simulink model "PPS_Model"  (Simulink 7.6)
settings: Solver=FixedStepDiscrete  SolverMode=SingleTasking  StartTime=0.0  StopTime=inf  FixedStep=1/100  RelTol=1e-3
undefined symbols (not defined in the file): dfreq, gray, nbboxout, Rec, SDTV, strel
libraries: simulink x21, viptextngfix x15, simulink_extras x3, vipconversions x3, vipsnks x2, vipstatistics x1, vipmorphops x1, vipanalysis x1
(part 1 of 2)
settings Model: Creator=Krzysztof  LastModifiedBy=MarcinB  BufferReuse=off
settings DataIOCC: SaveOutput=off  SaveTime=off
settings OptimizationCC: InlineParams=on  OptimizeBlockIOStorage=off  BufferReuse=off  ExpressionFolding=off  LocalBlockOutputs=off  SimCompilerOptimization=On
settings DebuggingCC: ReadBeforeWriteMsg=DisableAll  WriteAfterWriteMsg=DisableAll  WriteAfterReadMsg=DisableAll  SolverPrmCheckMsg=none  MultiTaskDSMMsg=none  SigSpecEnsureSampleTimeMsg=none  ParameterPrecisionLossMsg=none  UnknownTsInhSupMsg=none
settings ModelReferenceCC: ModelReferenceNumInstancesAllowed=Single
settings SFSimCC: SimParseCustomCode=off

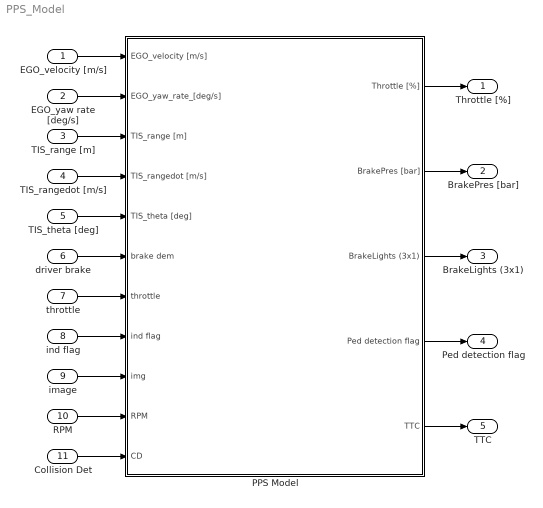
== system PPS_Model ==
  EGO_velocity [m/s] : Inport
  EGO_yaw rate [deg/s] : Inport  Port=2
  TIS_range [m] : Inport  Port=3
  TIS_rangedot [m/s] : Inport  Port=4
  TIS_theta [deg] : Inport  Port=5
  driver brake : Inport  Port=6
  throttle : Inport  Port=7
  ind flag : Inport  Port=8
  image : Inport  Port=9
  RPM : Inport  Port=10
  Collision Det : Inport  Port=11
  PPS Model : Subsystem  mask(PPS Model){MaxSpeed=70, MaxBrakePressure=150, BrakeDelay=100, LaneWidth=3.5, TISMaxRange=40, TISMaxTheta=60, TISfreq=25, TISdet=32, Camfreq=50, Mainfreq=100, DisplaySwitch=on, DisplayFreq=25, RadarSwitch=on, RadarFreq=25}
      mask prompts: MaxSpeed "Vehicle cut-off speed [km/h]"; MaxBrakePressure "Maximum value of braking pressure available [bar]"; BrakeDelay "Braking system delay [ms]"; LaneWidth "Lane width [m]"; TISMaxRange "TIS maximum range [m]"; TISMaxTheta "TIS maximum theta [deg]"; TISfreq "TIS frequency [Hz]"; TISdet "Max. number of Radar detected objects [-]"; Camfreq "Camera frequency [Hz]"; Mainfreq "Compilation sheet frequency [Hz]"; DisplaySwitch "Show EGO parameters visualization"; DisplayFreq "EGO parameters visualization frequency [Hz]"; RadarSwitch "Show radar visualization"; RadarFreq "Radar frequency [Hz]"
      mask help: PreScan Experiment and Pedestrian Protection System parameters
      mask Help: eval('openHelp(8130)')
      mask CallbackString:
      | ||||||||||en = get_param(gcb,'MaskEnables');
      | switch get_param(gcb, 'DisplaySwitch')
      |     case 'off'
      |         en{12} = 'off';
      |     case 'on'
      |         en{12} = 'on';
      | end
      | set_param(gcb,'MaskEnables',en);
      | clear en;||en = get_param(gcb,'MaskEnables');
      | switch get_param(gcb, 'RadarSwitch')
      |     case 'off'
      |         en{14} = 'off';
      |     case 'on'
      |         en{14} = 'on';
      | end
      | set_param(gcb,'MaskEnables',en);
      | clear en;|
  Throttle [%] : Outport
  BrakePres [bar] : Outport  Port=2
  BrakeLights (3x1) : Outport  Port=3
  Ped detection flag : Outport  Port=4
  TTC : Outport  Port=5
  wires:
  EGO_velocity [m/s]/1 -> PPS Model/1(EGO_velocity [m/s])
  EGO_yaw rate [deg/s]/1 -> PPS Model/2(EGO_yaw_rate_[deg/s])
  TIS_range [m]/1 -> PPS Model/3(TIS_range [m])
  TIS_rangedot [m/s]/1 -> PPS Model/4(TIS_rangedot [m/s])
  TIS_theta [deg]/1 -> PPS Model/5(TIS_theta [deg])
  throttle/1 -> PPS Model/7(throttle)
  ind flag/1 -> PPS Model/8(ind flag)
  image/1 -> PPS Model/9(img)
  PPS Model/1(Throttle [%]) -> Throttle [%]/1
  PPS Model/2(BrakePres [bar]) -> BrakePres [bar]/1
  PPS Model/3(BrakeLights (3x1)) -> BrakeLights (3x1)/1
  PPS Model/5(TTC) -> TTC/1
  driver brake/1 -> PPS Model/6(brake dem)
  RPM/1 -> PPS Model/10(RPM)
  Collision Det/1 -> PPS Model/11(CD)
  PPS Model/4(Ped detection flag) -> Ped detection flag/1

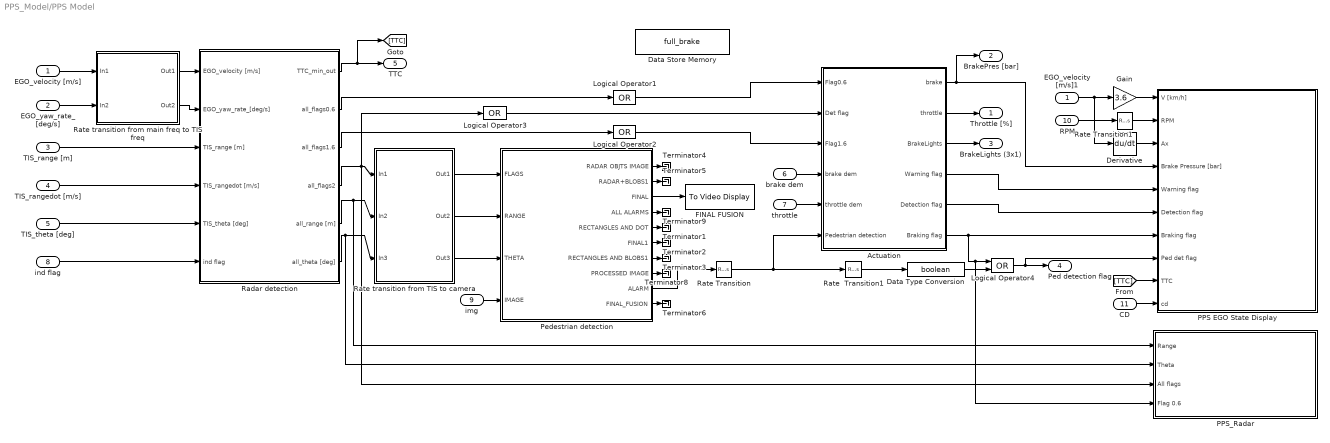
== system PPS_Model/PPS Model ==
  EGO_velocity [m/s] : Inport
  EGO_yaw_rate_[deg/s] : Inport  Port=2  SampleTime=1/Mainfreq
  TIS_range [m] : Inport  Port=3  PortDimensions=TISdet  SampleTime=1/TISfreq
  TIS_rangedot [m/s] : Inport  Port=4  PortDimensions=TISdet  SampleTime=1/TISfreq
  TIS_theta [deg] : Inport  Port=5  PortDimensions=TISdet  SampleTime=1/TISfreq
  brake dem : Inport  Port=6  SampleTime=[0,0]
  throttle : Inport  Port=7  SampleTime=[0,0]
  ind flag : Inport  Port=8  SampleTime=1/TISfreq
  img : Inport  Port=9  PortDimensions=[375 500]  SampleTime=1/Camfreq
  RPM : Inport  Port=10
  CD : Inport  Port=11
  Actuation : Subsystem
  Data Store Memory : DataStoreMemory  DataStoreName=full_brake  ReadBeforeWriteMsg=warning  WriteAfterWriteMsg=warning  WriteAfterReadMsg=warning
  Data Type Conversion : DataTypeConversion  OutDataTypeStr=boolean
  Derivative : Derivative
  EGO_velocity [m/s]1 : InportShadow  Port=1
  FINAL FUSION : vipsnks/To Video Display  DialogControllerArgs=DataTag0  inputType=Obsolete  imagePorts=One multidimensional signal  OutputDevice=On-screen video monitor  fullScreen=off  videoWindowX=530  videoWindowY=74  saveWindowSize=off  videoWindowWidth=500  videoWindowHeight=375  dataOrg=Column-major  openAtMdlStart=on  isWindowOpen=on
  Gain : Gain  Gain=3.6
  Logical Operator1 : Logic  Operator=OR  Inputs=1  AllPortsSameDT=off  OutDataTypeStr=boolean
  Logical Operator2 : Logic  Operator=OR  Inputs=1  AllPortsSameDT=off  OutDataTypeStr=boolean
  Logical Operator3 : Logic  Operator=OR  Inputs=1  AllPortsSameDT=off  OutDataTypeStr=boolean
  Logical Operator4 : Logic  Operator=OR  AllPortsSameDT=off  OutDataTypeStr=boolean
  PPS EGO State Display : Subsystem
  PPS_Radar : Subsystem
  Pedestrian detection : Subsystem
  Radar detection : Subsystem
  Rate  Transition1 : RateTransition  Integrity=off  Deterministic=off  OutPortSampleTime=1/min(TISfreq,Camfreq)
  Rate Transition : RateTransition  Integrity=off  Deterministic=off  OutPortSampleTime=[0,0]
  Rate Transition1 : RateTransition  Integrity=off  Deterministic=off  OutPortSampleTime=1/Mainfreq
  Rate transition from TIS to camera : Subsystem
  Rate transition from main freq to TIS freq : Subsystem
  Terminator{1..6,8..9} (8 alike) : Terminator
  Throttle [%] : Outport
  BrakePres [bar] : Outport  Port=2
  BrakeLights (3x1) : Outport  Port=3
  Ped detection flag : Outport  Port=4  PortDimensions=1
  TTC : Outport  Port=5
  wires:
  TIS_range [m]/1 -> Radar detection/3(TIS_range [m])
  TIS_rangedot [m/s]/1 -> Radar detection/4(TIS_rangedot [m/s])
  TIS_theta [deg]/1 -> Radar detection/5(TIS_theta [deg])
  ind flag/1 -> Radar detection/6(ind flag)
  EGO_velocity [m/s]/1 -> Rate transition from main freq to TIS freq/1(In1)
  EGO_yaw_rate_[deg/s]/1 -> Rate transition from main freq to TIS freq/2(In2)
  Rate transition from main freq to TIS freq/1(Out1) -> Radar detection/1(EGO_velocity [m/s])
  Rate transition from main freq to TIS freq/2(Out2) -> Radar detection/2(EGO_yaw_rate_[deg/s])
  throttle/1 -> Actuation/5(throttle dem)
  brake dem/1 -> Actuation/4(brake dem)
  Radar detection/1(TTC_min_out) -> TTC/1, [TTC]
  Radar detection/2(all_flags0.6) -> Logical Operator1/1
  Rate Transition/1 -> Actuation/6(Pedestrian detection), Rate  Transition1/1
  Rate  Transition1/1 -> Data Type Conversion/1
  Radar detection/4(all_flags2) -> Rate transition from TIS to camera/1(In1), Logical Operator3/1, PPS_Radar/3(All flags)
  Radar detection/5(all_range [m]) -> Rate transition from TIS to camera/2(In2), PPS_Radar/1(Range)
  Radar detection/6(all_theta [deg]) -> Rate transition from TIS to camera/3(In3), PPS_Radar/2(Theta)
  Radar detection/3(all_flags1.6) -> Logical Operator2/1
  Actuation/1(brake) -> BrakePres [bar]/1, PPS EGO State Display/4(Brake Pressure [bar])
  Actuation/2(throttle) -> Throttle [%]/1
  Actuation/3(BrakeLights) -> BrakeLights (3x1)/1
  Actuation/6(Braking flag) -> PPS EGO State Display/7(Braking flag), Logical Operator4/1, PPS_Radar/4(Flag 0.6)
  Pedestrian detection/8(PROCESSED IMAGE) -> Terminator8/1
  Pedestrian detection/4(ALL ALARMS) -> Terminator9/1
  Pedestrian detection/5(RECTANGLES AND DOT) -> Terminator1/1
  Pedestrian detection/7(RECTANGLES AND BLOBS1) -> Terminator3/1
  Pedestrian detection/2(RADAR+BLOBS1) -> Terminator5/1
  Pedestrian detection/1(RADAR OBJTS IMAGE) -> Terminator4/1
  Pedestrian detection/10(FINAL_FUSION) -> Terminator6/1
  img/1 -> Pedestrian detection/4(IMAGE)
  Pedestrian detection/3(FINAL) -> FINAL FUSION/1
  Pedestrian detection/9(ALARM) -> Rate Transition/1
  Pedestrian detection/6(FINAL1) -> Terminator2/1
  Rate transition from TIS to camera/1(Out1) -> Pedestrian detection/1(FLAGS)
  Rate transition from TIS to camera/2(Out2) -> Pedestrian detection/2(RANGE)
  Rate transition from TIS to camera/3(Out3) -> Pedestrian detection/3(THETA)
  Logical Operator1/1 -> Actuation/1(Flag0.6)
  Logical Operator2/1 -> Actuation/3(Flag1.6)
  Data Type Conversion/1 -> Logical Operator4/2
  Logical Operator4/1 -> Ped detection flag/1, PPS EGO State Display/8(Ped det flag)
  Logical Operator3/1 -> Actuation/2(Det flag)
  EGO_velocity [m/s]1/1 -> Gain/1, Derivative/1
  Gain/1 -> PPS EGO State Display/1(V [km/h])
  RPM/1 -> Rate Transition1/1
  Derivative/1 -> PPS EGO State Display/3(Ax)
  CD/1 -> PPS EGO State Display/10(cd)
  [TTC] -> PPS EGO State Display/9(TTC)
  Actuation/4(Warning flag) -> PPS EGO State Display/5(Warning flag)
  Actuation/5(Detection flag) -> PPS EGO State Display/6(Detection flag)
  Rate Transition1/1 -> PPS EGO State Display/2(RPM)

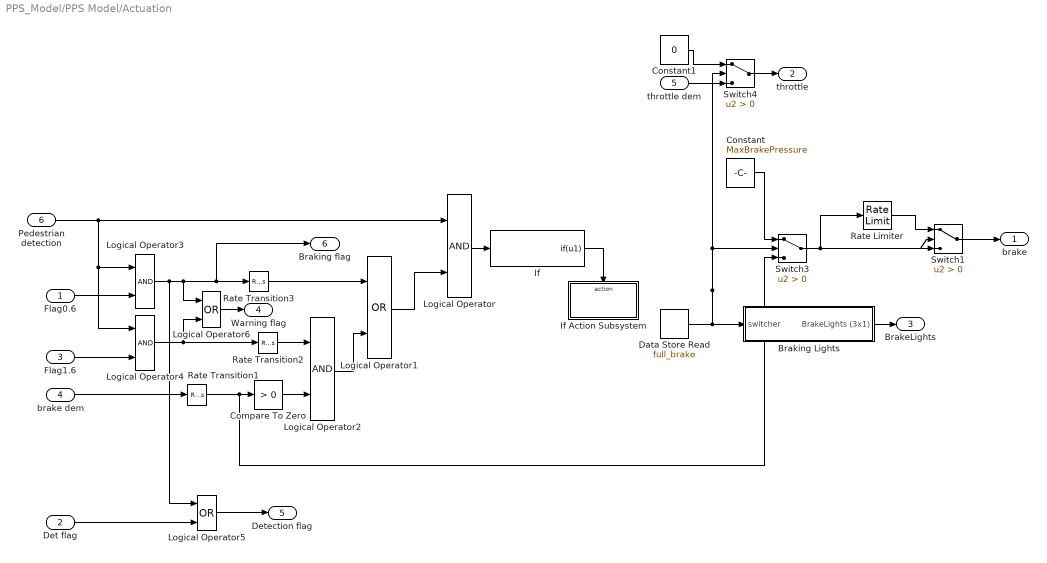
== system PPS_Model/PPS Model/Actuation ==
  Flag0.6 : Inport
  Det flag : Inport  Port=2
  Flag1.6 : Inport  Port=3
  brake dem : Inport  Port=4
  throttle dem : Inport  Port=5
  Pedestrian detection : Inport  Port=6
  Braking Lights : Subsystem
  Compare To Zero : simulink/Logic and Bit Operations/Compare To Zero  SystemSampleTime=-1  relop=>  LogicOutDataTypeMode=uint8
  Constant : Constant  Value=MaxBrakePressure  SampleTime=[0,0]
  Constant1 : Constant  Value=0  SampleTime=[0,0]
  Data Store Read : DataStoreRead  DataStoreName=full_brake  SampleTime=1/Mainfreq
  If : If  IfExpression=u1  ShowElse=off
  If Action Subsystem : Subsystem  TreatAsAtomicUnit=on
  Logical Operator : Logic  AllPortsSameDT=off  OutDataTypeStr=boolean  SampleTime=[0,0]
  Logical Operator1 : Logic  Operator=OR  AllPortsSameDT=off  OutDataTypeStr=boolean  SampleTime=[0,0]
  Logical Operator2 : Logic  AllPortsSameDT=off  OutDataTypeStr=boolean  SampleTime=[0,0]
  Logical Operator3 : Logic  AllPortsSameDT=off  OutDataTypeStr=boolean  SampleTime=1/TISfreq
  Logical Operator4 : Logic  AllPortsSameDT=off  OutDataTypeStr=boolean  SampleTime=1/TISfreq
  Logical Operator5 : Logic  Operator=OR  AllPortsSameDT=off  OutDataTypeStr=boolean  SampleTime=1/TISfreq
  Logical Operator6 : Logic  Operator=OR  AllPortsSameDT=off  OutDataTypeStr=boolean  SampleTime=1/TISfreq
  Rate Limiter : RateLimiter  RisingSlewLimit=1000*0.9*MaxBrakePressure/BrakeDelay  FallingSlewLimit=-inf  SampleTimeMode=inherited
  Rate Transition1 : RateTransition  Integrity=off  OutPortSampleTime=[0,0]
  Rate Transition2 : RateTransition  Integrity=off  OutPortSampleTime=[0,0]
  Rate Transition3 : RateTransition  Integrity=off  OutPortSampleTime=[0,0]
  Switch1 : Switch  Criteria=u2 > Threshold  SampleTime=[0,0]
  Switch3 : Switch  Criteria=u2 > Threshold  SampleTime=[0,0]
  Switch4 : Switch  Criteria=u2 > Threshold  SampleTime=[0,0]
  brake : Outport  SampleTime=[0,0]
  throttle : Outport  Port=2  SampleTime=[0,0]
  BrakeLights : Outport  Port=3  SampleTime=1/Mainfreq
  Warning flag : Outport  Port=4
  Detection flag : Outport  Port=5
  Braking flag : Outport  Port=6
  wires:
  Pedestrian detection/1 -> Logical Operator3/1, Logical Operator4/1, Logical Operator/1
  Logical Operator1/1 -> Logical Operator/2
  Logical Operator2/1 -> Logical Operator1/2
  Compare To Zero/1 -> Logical Operator2/2
  Constant/1 -> Switch3/1
  Constant1/1 -> Switch4/1
  Switch4/1 -> throttle/1
  throttle dem/1 -> Switch4/3
  Braking Lights/1(BrakeLights (3x1)) -> BrakeLights/1
  brake dem/1 -> Rate Transition1/1
  Rate Transition1/1 -> Compare To Zero/1, Switch3/3
  Rate Transition2/1 -> Logical Operator2/1
  Rate Transition3/1 -> Logical Operator1/1
  Switch3/1 -> Switch1/3, Rate Limiter/1
  Rate Limiter/1 -> Switch1/1
  Switch1/1 -> brake/1
  Logical Operator3/1 -> Rate Transition3/1, Braking flag/1, Logical Operator6/1, Logical Operator5/1
  Logical Operator4/1 -> Rate Transition2/1, Logical Operator6/2
  Flag0.6/1 -> Logical Operator3/2
  Flag1.6/1 -> Logical Operator4/2
  Logical Operator6/1 -> Warning flag/1
  Det flag/1 -> Logical Operator5/2
  Logical Operator5/1 -> Detection flag/1
  Logical Operator/1 -> If/1
  Data Store Read/1 -> Braking Lights/1(switcher), Switch3/2, Switch1/2, Switch4/2
  If/1 -> If Action Subsystem/Action

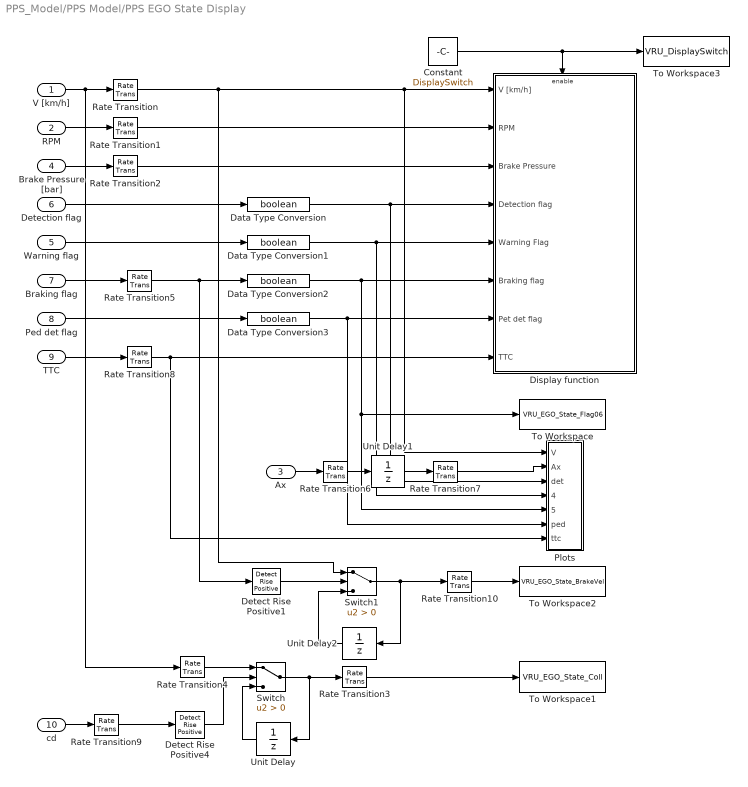
== system PPS_Model/PPS Model/PPS EGO State Display ==
  V [km/h] : Inport
  RPM : Inport  Port=2
  Ax : Inport  Port=3  SampleTime=[0,0]
  Brake Pressure [bar] : Inport  Port=4
  Warning flag : Inport  Port=5  OutDataTypeStr=boolean
  Detection flag : Inport  Port=6  OutDataTypeStr=boolean
  Braking flag : Inport  Port=7  OutDataTypeStr=boolean
  Ped det flag : Inport  Port=8  OutDataTypeStr=boolean
  TTC : Inport  Port=9
  cd : Inport  Port=10  OutDataTypeStr=boolean
  Constant : Constant  Value=DisplaySwitch
  Data Type Conversion{,1..3} (4 alike) : DataTypeConversion  OutDataTypeStr=boolean
  Detect Rise Positive1 : simulink/Logic and Bit Operations/Detect Rise Positive  SystemSampleTime=-1  vinit=0
  Detect Rise Positive4 : simulink/Logic and Bit Operations/Detect Rise Positive  SystemSampleTime=-1  vinit=0
  Display function : Subsystem
  Plots : Subsystem
      mask Description:
      | The block calls functions:
      | * PPS_Speed_Profile
      | * PPS_TTC_Profile
      | to generate plots at the end of the simulation.
      | See stop callback of the block for more details.
  Rate Transition{,1..2,5,7..8} (6 alike) : RateTransition  Integrity=off  OutPortSampleTime=1/DisplayFreq
  Rate Transition10 : RateTransition  Integrity=off  OutPortSampleTime=[0,0]
  Rate Transition3 : RateTransition  Integrity=off  OutPortSampleTime=[0,0]
  Rate Transition4 : RateTransition  Integrity=off  OutPortSampleTime=1/Mainfreq
  Rate Transition6 : RateTransition  Integrity=off  OutPortSampleTimeOpt=Inherit  OutPortSampleTime=1/dfreq
  Rate Transition9 : RateTransition  Integrity=off  OutPortSampleTime=1/Mainfreq
  Switch : Switch  Criteria=u2 > Threshold  SampleTime=1/Mainfreq
  Switch1 : Switch  Criteria=u2 > Threshold  SampleTime=1/Mainfreq
  To Workspace : ToWorkspace  VariableName=VRU_EGO_State_Flag06  SampleTime=-1  SaveFormat=Array
      settings: MaxDataPoints=1
  To Workspace1 : ToWorkspace  VariableName=VRU_EGO_State_Coll  SampleTime=1/Mainfreq  SaveFormat=Array
      settings: MaxDataPoints=1
  To Workspace2 : ToWorkspace  VariableName=VRU_EGO_State_BrakeVel  SampleTime=1/Mainfreq  SaveFormat=Array
      settings: MaxDataPoints=1
  To Workspace3 : ToWorkspace  VariableName=VRU_DisplaySwitch  SampleTime=-1  SaveFormat=Array
      settings: MaxDataPoints=1
  Unit Delay : UnitDelay  SampleTime=1/Mainfreq
  Unit Delay1 : UnitDelay  SampleTime=-1
  Unit Delay2 : UnitDelay  SampleTime=1/Mainfreq
  wires:
  RPM/1 -> Rate Transition1/1
  Brake Pressure [bar]/1 -> Rate Transition2/1
  V [km/h]/1 -> Rate Transition/1, Rate Transition4/1
  Warning flag/1 -> Data Type Conversion1/1
  Ped det flag/1 -> Data Type Conversion3/1
  TTC/1 -> Rate Transition8/1
  Detection flag/1 -> Data Type Conversion/1
  Rate Transition/1 -> Display function/1(V [km/h]), Plots/1(V), Switch1/1
  Rate Transition1/1 -> Display function/2(RPM)
  Rate Transition3/1 -> To Workspace1/1
  cd/1 -> Rate Transition9/1
  Switch/1 -> Unit Delay/1, Rate Transition3/1
  Unit Delay/1 -> Switch/3
  Rate Transition4/1 -> Switch/1
  Detect Rise Positive4/1 -> Switch/2
  Braking flag/1 -> Rate Transition5/1
  Rate Transition5/1 -> Data Type Conversion2/1, Detect Rise Positive1/1
  Ax/1 -> Rate Transition6/1
  Unit Delay1/1 -> Rate Transition7/1
  Rate Transition6/1 -> Unit Delay1/1
  Rate Transition2/1 -> Display function/3(Brake Pressure)
  Rate Transition7/1 -> Plots/2(Ax)
  Rate Transition8/1 -> Plots/7(ttc), Display function/8(TTC)
  Rate Transition9/1 -> Detect Rise Positive4/1
  Data Type Conversion3/1 -> Plots/6(ped), Display function/7(Pet det flag)
  Data Type Conversion2/1 -> Plots/5(brake), To Workspace/1, Display function/6(Braking flag)
  Data Type Conversion1/1 -> Plots/4(warn), Display function/5(Warning Flag)
  Data Type Conversion/1 -> Plots/3(det), Display function/4(Detection flag)
  Constant/1 -> Display function/Enable, To Workspace3/1
  Detect Rise Positive1/1 -> Switch1/2
  Switch1/1 -> Unit Delay2/1, Rate Transition10/1
  Unit Delay2/1 -> Switch1/3
  Rate Transition10/1 -> To Workspace2/1

== system PPS_Model/PPS Model/PPS_Radar ==
  Range : Inport
  Theta : Inport  Port=2
  All flags : Inport  Port=3  OutDataTypeStr=boolean
  Flag 0.6 : Inport  Port=4  OutDataTypeStr=boolean
  Constant : Constant  Value=RadarSwitch
  Radar : Subsystem
  Rate Transition{1..4} (4 alike) : RateTransition  Integrity=off  Deterministic=off  OutPortSampleTime=1/RadarFreq
  wires:
  Range/1 -> Rate Transition1/1
  Theta/1 -> Rate Transition2/1
  All flags/1 -> Rate Transition3/1
  Flag 0.6/1 -> Rate Transition4/1
  Rate Transition1/1 -> Radar/1(Range)
  Rate Transition2/1 -> Radar/2(Theta)
  Rate Transition3/1 -> Radar/3(All flags)
  Rate Transition4/1 -> Radar/4(Flag 0.6)
  Constant/1 -> Radar/Enable

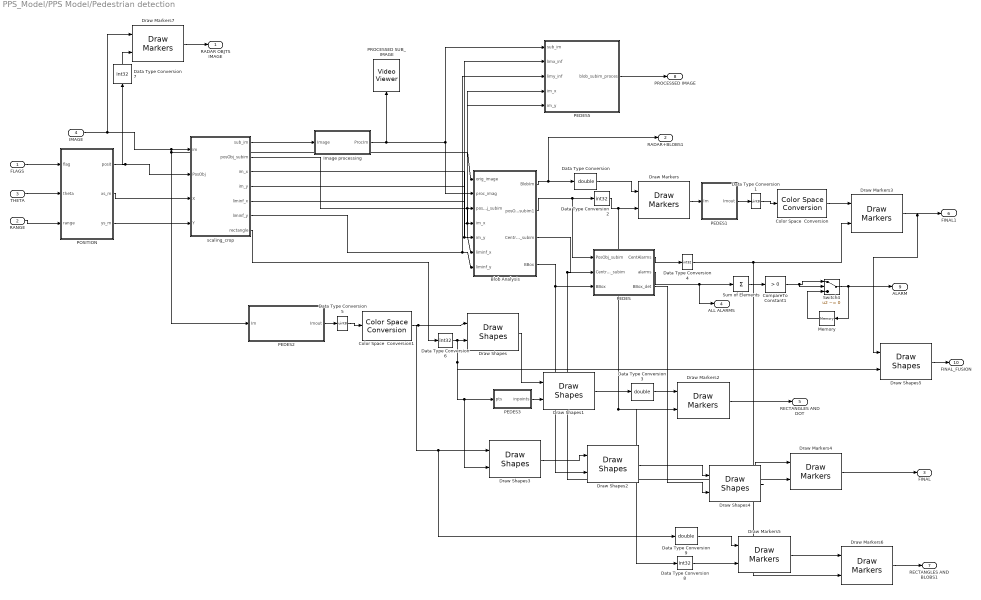
== system PPS_Model/PPS Model/Pedestrian detection ==
  FLAGS : Inport  OutDataTypeStr=boolean
  RANGE : Inport  Port=2  PortDimensions=TISdet
  THETA : Inport  Port=3
  IMAGE : Inport  Port=4  OutDataTypeStr=uint8  PortDimensions=[375 500]
  Blob Analysis : Subsystem
  Color Space  Conversion : vipconversions/Color Space  Conversion  conversion=Obsolete  conversionActive=Y'CbCr to R'G'B'  wp_str=D65  rec=Rec. 601 (SDTV)  sys=1125/60/2:1  imagePorts=One multidimensional signal
  Color Space  Conversion1 : vipconversions/Color Space  Conversion  conversion=Obsolete  conversionActive=Y'CbCr to R'G'B'  wp_str=D65  rec=Rec. 601 (SDTV)  sys=1125/60/2:1  imagePorts=One multidimensional signal
  CompareTo Constant1 : simulink/Logic and Bit Operations/Compare To Constant  SystemSampleTime=-1  relop=>  const=0  LogicOutDataTypeMode=uint8
  Data Type Conversion : DataTypeConversion  OutDataTypeStr=double
  Data Type Conversion1 : DataTypeConversion  OutDataTypeStr=uint8
  Data Type Conversion{2,4,6..8} (5 alike) : DataTypeConversion  OutDataTypeStr=int32
  Data Type Conversion3 : DataTypeConversion  OutDataTypeStr=double
  Data Type Conversion5 : DataTypeConversion  OutDataTypeStr=uint8
  Data Type Conversion9 : DataTypeConversion  OutDataTypeStr=double
  Draw Markers : viptextngfix/Draw Markers  DialogController=vipDDGCreate  DialogControllerArgs=DataTag4  shape=Circle  size=6  fill=on  fillClrSource=Specify via dialog  display=White  intensity=200  color=[200 255 100]  opacity=0.9  viewport=Entire image  antialiasing=on  inType=Obsolete  imagePorts=One multidimensional signal  prodOutputMode=Binary point scaling  prodOutputWordLength=32  prodOutputFracLength=14  memoryMode=Specify word length  memoryWordLength=16  memoryFracLength=14  roundingMode=Floor  overflowMode=off
  Draw Markers2 : viptextngfix/Draw Markers  DialogController=vipDDGCreate  DialogControllerArgs=DataTag5  shape=Circle  size=6  fill=on  fillClrSource=Specify via dialog  display=White  intensity=200  color=[200 255 100]  opacity=0.9  viewport=Entire image  antialiasing=on  inType=Obsolete  imagePorts=One multidimensional signal  prodOutputMode=Binary point scaling  prodOutputWordLength=32  prodOutputFracLength=14  memoryMode=Specify word length  memoryWordLength=16  memoryFracLength=14  roundingMode=Floor  overflowMode=off
  Draw Markers3 : viptextngfix/Draw Markers  DialogController=vipDDGCreate  DialogControllerArgs=DataTag6  shape=Circle  size=6  fill=on  fillClrSource=Specify via dialog  display=User-specified value  intensity=200  color=[255 0 0]  opacity=1  viewport=Entire image  antialiasing=on  inType=Obsolete  imagePorts=One multidimensional signal  prodOutputMode=Binary point scaling  prodOutputWordLength=32  prodOutputFracLength=14  memoryMode=Specify word length  memoryWordLength=16  memoryFracLength=14  roundingMode=Floor  overflowMode=off
  Draw Markers4 : viptextngfix/Draw Markers  DialogController=vipDDGCreate  DialogControllerArgs=DataTag7  shape=X-mark  size=3  fill=on  fillClrSource=Specify via dialog  display=White  intensity=200  color=[200 255 100]  opacity=0.9  viewport=Entire image  antialiasing=on  inType=Obsolete  imagePorts=One multidimensional signal  prodOutputMode=Binary point scaling  prodOutputWordLength=32  prodOutputFracLength=14  memoryMode=Specify word length  memoryWordLength=16  memoryFracLength=14  roundingMode=Floor  overflowMode=off
  Draw Markers5 : viptextngfix/Draw Markers  DialogController=vipDDGCreate  DialogControllerArgs=DataTag8  shape=Circle  size=6  fill=on  fillClrSource=Specify via dialog  display=White  intensity=200  color=[200 255 100]  opacity=0.9  viewport=Entire image  antialiasing=on  inType=Obsolete  imagePorts=One multidimensional signal  prodOutputMode=Binary point scaling  prodOutputWordLength=32  prodOutputFracLength=14  memoryMode=Specify word length  memoryWordLength=16  memoryFracLength=14  roundingMode=Floor  overflowMode=off
  Draw Markers6 : viptextngfix/Draw Markers  DialogController=vipDDGCreate  DialogControllerArgs=DataTag9  shape=Circle  size=6  fill=on  fillClrSource=Specify via dialog  display=User-specified value  intensity=200  color=[255 0 0]  opacity=1  viewport=Entire image  antialiasing=on  inType=Obsolete  imagePorts=One multidimensional signal  prodOutputMode=Binary point scaling  prodOutputWordLength=32  prodOutputFracLength=14  memoryMode=Specify word length  memoryWordLength=16  memoryFracLength=14  roundingMode=Floor  overflowMode=off
  Draw Markers7 : viptextngfix/Draw Markers  DialogController=vipDDGCreate  DialogControllerArgs=DataTag10  shape=Circle  size=6  fill=on  fillClrSource=Specify via dialog  display=White  intensity=200  color=[200 255 100]  opacity=1  viewport=Entire image  antialiasing=on  inType=Obsolete  imagePorts=One multidimensional signal  prodOutputMode=Binary point scaling  prodOutputWordLength=32  prodOutputFracLength=14  memoryMode=Specify word length  memoryWordLength=16  memoryFracLength=14  roundingMode=Floor  overflowMode=off
  Draw Shapes : viptextngfix/Draw Shapes  DialogController=vipDDGCreate  DialogControllerArgs=DataTag11  shape=Rectangles  fill=off  fillClrSource=Specify via dialog  display=User-specified value  intensity=200  color=[255 0 0]  opacity=0.5  viewport=Entire image  antialiasing=off  inType=Obsolete  imagePorts=One multidimensional signal  prodOutputMode=Binary point scaling  prodOutputWordLength=32  prodOutputFracLength=14  memoryMode=Specify word length  memoryWordLength=16  memoryFracLength=14  roundingMode=Floor  overflowMode=off
  Draw Shapes1 : viptextngfix/Draw Shapes  DialogController=vipDDGCreate  DialogControllerArgs=DataTag12  shape=Rectangles  fill=on  fillClrSource=Specify via dialog  display=White  intensity=200  color=[255 0 0]  opacity=0.5  viewport=Entire image  antialiasing=off  inType=Obsolete  imagePorts=One multidimensional signal  prodOutputMode=Binary point scaling  prodOutputWordLength=32  prodOutputFracLength=14  memoryMode=Specify word length  memoryWordLength=16  memoryFracLength=14  roundingMode=Floor  overflowMode=off
  Draw Shapes2 : viptextngfix/Draw Shapes  DialogController=vipDDGCreate  DialogControllerArgs=DataTag13  shape=Rectangles  fill=off  fillClrSource=Specify via dialog  display=User-specified value  intensity=200  color=[255 0 0]  opacity=0.6  viewport=Entire image  antialiasing=off  inType=Obsolete  imagePorts=One multidimensional signal  prodOutputMode=Binary point scaling  prodOutputWordLength=32  prodOutputFracLength=14  memoryMode=Specify word length  memoryWordLength=16  memoryFracLength=14  roundingMode=Floor  overflowMode=off
  Draw Shapes3 : viptextngfix/Draw Shapes  DialogController=vipDDGCreate  DialogControllerArgs=DataTag14  shape=Rectangles  fill=off  fillClrSource=Specify via dialog  display=White  intensity=200  color=[255 0 0]  opacity=0.5  viewport=Entire image  antialiasing=off  inType=Obsolete  imagePorts=One multidimensional signal  prodOutputMode=Binary point scaling  prodOutputWordLength=32  prodOutputFracLength=14  memoryMode=Specify word length  memoryWordLength=16  memoryFracLength=14  roundingMode=Floor  overflowMode=off
  Draw Shapes4 : viptextngfix/Draw Shapes  DialogController=vipDDGCreate  DialogControllerArgs=DataTag15  shape=Rectangles  fill=on  fillClrSource=Specify via dialog  display=White  intensity=200  color=[255 0 0]  opacity=0.5  viewport=Entire image  antialiasing=off  inType=Obsolete  imagePorts=One multidimensional signal  prodOutputMode=Binary point scaling  prodOutputWordLength=32  prodOutputFracLength=14  memoryMode=Specify word length  memoryWordLength=16  memoryFracLength=14  roundingMode=Floor  overflowMode=off
  Draw Shapes5 : viptextngfix/Draw Shapes  DialogController=vipDDGCreate  DialogControllerArgs=DataTag16  shape=Rectangles  fill=off  fillClrSource=Specify via dialog  display=White  intensity=200  color=[255 0 0]  opacity=0.6  viewport=Entire image  antialiasing=off  inType=Obsolete  imagePorts=One multidimensional signal  prodOutputMode=Binary point scaling  prodOutputWordLength=32  prodOutputFracLength=14  memoryMode=Specify word length  memoryWordLength=16  memoryFracLength=14  roundingMode=Floor  overflowMode=off
  Image processing : Subsystem
  Memory : Memory
  PEDES : Stateflow chart  TreatAsAtomicUnit=on
  PEDES1 : Stateflow chart  TreatAsAtomicUnit=on
  PEDES2 : Stateflow chart  TreatAsAtomicUnit=on
  PEDES3 : Stateflow chart  TreatAsAtomicUnit=on
  PEDES5 : Stateflow chart  TreatAsAtomicUnit=on
  POSITION : Stateflow chart  TreatAsAtomicUnit=on
  PROCESSED SUB_IMAGE : vipsnks/Video Viewer  DialogControllerArgs=DataTag19  inputType=Obsolete7b  imagePorts=One multidimensional signal  useColorMap=off  colormapValue=gray(256)  specRange=off  minInputVal=0  maxInputVal=255  FigPos=[546 1020 501 324]  AxisZoom=on  trueSizedOnce=off  OpenAtMdlStart=on
  Sum of Elements : Sum  Inputs=+
  Switch4 : Switch  Criteria=u2 ~= 0
  scaling_crop : Stateflow chart  TreatAsAtomicUnit=on
  RADAR OBJTS IMAGE : Outport
  RADAR+BLOBS1 : Outport  Port=2
  FINAL : Outport  Port=3
  ALL ALARMS : Outport  Port=4
  RECTANGLES AND DOT : Outport  Port=5
  FINAL1 : Outport  Port=6
  RECTANGLES AND BLOBS1 : Outport  Port=7
  PROCESSED IMAGE : Outport  Port=8
  ALARM : Outport  Port=9
  FINAL_FUSION : Outport  Port=10
  wires:
  THETA/1 -> POSITION/2(theta)
  FLAGS/1 -> POSITION/1(flag)
  RANGE/1 -> POSITION/3(range)
  Blob Analysis/1(BlobIm) -> RADAR+BLOBS1/1, Data Type Conversion/1
  Blob Analysis/3(Centroid_subim) -> PEDES/2(Centroid_subim), Draw Markers4/2
  PEDES/2(alarms) -> ALL ALARMS/1, Sum of Elements/1
  PEDES/1(CentAlarms) -> Data Type Conversion4/1
  Blob Analysis/4(BBox) -> PEDES/3(BBox), Draw Shapes2/2
  Draw Markers/1 -> PEDES1/1(Im)
  Data Type Conversion4/1 -> Draw Markers3/2, Draw Markers6/2
  Color Space  Conversion/1 -> Draw Markers3/1
  PEDES1/1(Imout) -> Data Type Conversion1/1
  Data Type Conversion1/1 -> Color Space  Conversion/1
  Data Type Conversion2/1 -> Draw Markers/2, Draw Markers2/2, Data Type Conversion8/1
  Switch4/1 -> Memory/1, ALARM/1
  Memory/1 -> Switch4/3
  Sum of Elements/1 -> CompareTo Constant1/1
  CompareTo Constant1/1 -> Switch4/1, Switch4/2
  Blob Analysis/2(posObj_subim1) -> Data Type Conversion2/1, PEDES/1(PosObj_subim)
  scaling_crop/6(liminf_y) -> Blob Analysis/7(liminf_y), PEDES5/3(limy_inf)
  scaling_crop/7(rectangle) -> Data Type Conversion6/1
  PEDES2/1(Imout) -> Data Type Conversion5/1
  Data Type Conversion5/1 -> Color Space  Conversion1/1
  Color Space  Conversion1/1 -> Draw Shapes3/1, Data Type Conversion9/1, Draw Shapes/1
  Data Type Conversion6/1 -> Draw Shapes/2, Draw Shapes3/2, PEDES3/1(pts), Draw Shapes5/2
  Draw Shapes/1 -> Draw Shapes1/1
  Draw Shapes1/1 -> Data Type Conversion3/1
  Draw Markers2/1 -> RECTANGLES AND DOT/1
  Draw Shapes3/1 -> Draw Shapes2/1
  Draw Shapes2/1 -> Draw Shapes4/1
  Draw Shapes4/1 -> Draw Markers4/1
  Draw Markers5/1 -> Draw Markers6/1
  Data Type Conversion8/1 -> Draw Markers5/2
  Draw Markers6/1 -> RECTANGLES AND BLOBS1/1
  PEDES3/1(inpoints) -> Draw Shapes1/2
  PEDES5/1(blob_subim_proces) -> PROCESSED IMAGE/1
  Draw Markers3/1 -> Draw Shapes5/1, FINAL1/1
  Draw Shapes5/1 -> FINAL_FUSION/1
  Data Type Conversion7/1 -> Draw Markers7/2
  POSITION/2(xs_m) -> scaling_crop/3(X)
  Draw Markers7/1 -> RADAR OBJTS IMAGE/1
  POSITION/3(ys_m) -> scaling_crop/4(Y)
  POSITION/1(posit) -> scaling_crop/2(PosObj), Data Type Conversion7/1
  IMAGE/1 -> Draw Markers7/1, scaling_crop/1(im), PEDES2/1(Im), Blob Analysis/1(orig_image)
  scaling_crop/1(sub_im) -> Image processing/1(Image)
  scaling_crop/2(posObj_subim) -> Blob Analysis/3(posObj_subim)
  scaling_crop/3(im_x) -> Blob Analysis/4(im_x), PEDES5/4(im_x)
  scaling_crop/4(im_y) -> Blob Analysis/5(im_y), PEDES5/5(im_y)
  scaling_crop/5(liminf_x) -> Blob Analysis/6(liminf_x), PEDES5/2(limx_inf)
  PEDES/3(BBox_det) -> Draw Shapes4/2
  Draw Markers4/1 -> FINAL/1
  Image processing/1(ProcIm) -> PEDES5/1(sub_im), Blob Analysis/2(proc_imag), PROCESSED SUB_IMAGE/1
  Data Type Conversion/1 -> Draw Markers/1
  Data Type Conversion9/1 -> Draw Markers5/1
  Data Type Conversion3/1 -> Draw Markers2/1

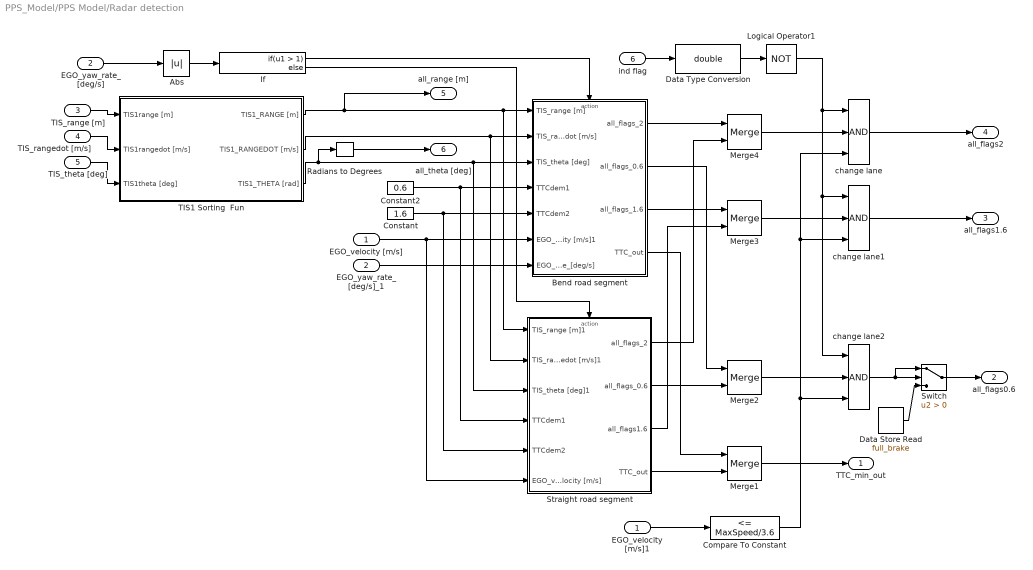
== system PPS_Model/PPS Model/Radar detection ==
  EGO_velocity [m/s] : Inport
  EGO_yaw_rate_[deg/s] : Inport  Port=2
  TIS_range [m] : Inport  Port=3  PortDimensions=TISdet
  TIS_rangedot [m/s] : Inport  Port=4  PortDimensions=TISdet
  TIS_theta [deg] : Inport  Port=5  PortDimensions=TISdet
  ind flag : Inport  Port=6
  Abs : Abs
  Bend road segment : Subsystem  TreatAsAtomicUnit=on
  Compare To Constant : simulink/Logic and Bit Operations/Compare To Constant  SystemSampleTime=-1  relop=<=  const=MaxSpeed/3.6  LogicOutDataTypeMode=uint8
  Constant : Constant  Value=1.6
  Constant2 : Constant  Value=0.6
  Data Store Read : DataStoreRead  DataStoreName=full_brake  SampleTime=1/Mainfreq
  Data Type Conversion : DataTypeConversion  OutDataTypeStr=double
  EGO_velocity [m/s]1 : InportShadow  Port=1
  EGO_yaw_rate_[deg/s]_1 : InportShadow  Port=2
  If : If  IfExpression=u1 > 1  SampleTime=1/TISfreq
  Logical Operator1 : Logic  Operator=NOT  AllPortsSameDT=off  OutDataTypeStr=boolean
  Merge{1..4} (4 alike) : Merge
  Radians to Degrees : simulink_extras/Transformations/Radians to Degrees  SystemSampleTime=-1
  Straight road segment : Subsystem  TreatAsAtomicUnit=on
  Switch : Switch  Criteria=u2 > Threshold
  TIS1 Sorting  Fun : Subsystem
  change lane : Logic  Inputs=3  AllPortsSameDT=off  OutDataTypeStr=boolean
  change lane1 : Logic  Inputs=3  AllPortsSameDT=off  OutDataTypeStr=boolean
  change lane2 : Logic  Inputs=3  AllPortsSameDT=off  OutDataTypeStr=boolean
  TTC_min_out : Outport
  all_flags0.6 : Outport  Port=2
  all_flags1.6 : Outport  Port=3
  all_flags2 : Outport  Port=4
  all_range [m] : Outport  Port=5
  all_theta [deg] : Outport  Port=6
  wires:
  TIS_range [m]/1 -> TIS1 Sorting  Fun/1(TIS1range [m])
  TIS_rangedot [m/s]/1 -> TIS1 Sorting  Fun/2(TIS1rangedot [m/s])
  TIS_theta [deg]/1 -> TIS1 Sorting  Fun/3(TIS1theta [deg])
  EGO_yaw_rate_[deg/s]/1 -> Abs/1
  If/1 -> Bend road segment/Action
  Abs/1 -> If/1
  TIS1 Sorting  Fun/1(TIS1_RANGE [m]) -> Bend road segment/1(TIS_range [m]), Straight road segment/1(TIS_range [m]1), all_range [m]/1
  TIS1 Sorting  Fun/2(TIS1_RANGEDOT [m/s]) -> Bend road segment/2(TIS_rangedot [m/s]), Straight road segment/2(TIS_rangedot [m/s]1)
  TIS1 Sorting  Fun/3(TIS1_THETA [rad]) -> Bend road segment/3(TIS_theta [deg]), Straight road segment/3(TIS_theta [deg]1), Radians to Degrees/1
  If/2 -> Straight road segment/Action
  Constant2/1 -> Bend road segment/4(TTCdem1), Straight road segment/4(TTCdem1)
  Constant/1 -> Bend road segment/5(TTCdem2), Straight road segment/5(TTCdem2)
  EGO_velocity [m/s]/1 -> Bend road segment/6(EGO_velocity [m/s]1), Straight road segment/6(EGO_velocity [m/s])
  EGO_yaw_rate_[deg/s]_1/1 -> Bend road segment/7(EGO_yaw_rate_[deg/s])
  ind flag/1 -> Data Type Conversion/1
  Bend road segment/2(all_flags_0.6) -> Merge2/1
  Straight road segment/2(all_flags_0.6) -> Merge2/2
  Straight road segment/3(all_flags1.6) -> Merge3/2
  Bend road segment/3(all_flags_1.6) -> Merge3/1
  Radians to Degrees/1 -> all_theta [deg]/1
  Data Type Conversion/1 -> Logical Operator1/1
  Straight road segment/4(TTC_out) -> Merge1/2
  Bend road segment/4(TTC_out) -> Merge1/1
  Merge1/1 -> TTC_min_out/1
  Bend road segment/1(all_flags_2) -> Merge4/1
  Straight road segment/1(all_flags_2) -> Merge4/2
  Merge4/1 -> change lane/2
  Logical Operator1/1 -> change lane/1, change lane2/1, change lane1/1
  Merge3/1 -> change lane1/2
  Merge2/1 -> change lane2/2
  change lane/1 -> all_flags2/1
  change lane2/1 -> Switch/2, Switch/1
  Switch/1 -> all_flags0.6/1
  EGO_velocity [m/s]1/1 -> Compare To Constant/1
  Compare To Constant/1 -> change lane2/3, change lane1/3, change lane/3
  change lane1/1 -> all_flags1.6/1
  Data Store Read/1 -> Switch/3

== system PPS_Model/PPS Model/Rate transition from TIS to camera ==
  In1 : Inport
  In2 : Inport  Port=2
  In3 : Inport  Port=3
  Rate Transition1 : RateTransition  Integrity=off  Deterministic=off  X0=zeros(TISdet,1)  OutPortSampleTime=1/Camfreq
  Rate Transition2 : RateTransition  Integrity=off  Deterministic=off  X0=zeros(TISdet,1)  OutPortSampleTime=1/Camfreq
  Rate Transition3 : RateTransition  Integrity=off  Deterministic=off  X0=zeros(TISdet,1)  OutPortSampleTime=1/Camfreq
  Out1 : Outport
  Out2 : Outport  Port=2
  Out3 : Outport  Port=3
  wires:
  In1/1 -> Rate Transition3/1
  In2/1 -> Rate Transition1/1
  In3/1 -> Rate Transition2/1
  Rate Transition3/1 -> Out1/1
  Rate Transition1/1 -> Out2/1
  Rate Transition2/1 -> Out3/1

== system PPS_Model/PPS Model/Rate transition from main freq to TIS freq ==
  In1 : Inport
  In2 : Inport  Port=2
  Rate Transition1 : RateTransition  Integrity=off  Deterministic=off  OutPortSampleTime=1/TISfreq
  Rate Transition2 : RateTransition  Integrity=off  Deterministic=off  OutPortSampleTime=1/TISfreq
  Out1 : Outport
  Out2 : Outport  Port=2
  wires:
  Rate Transition1/1 -> Out2/1
  In2/1 -> Rate Transition1/1
  In1/1 -> Rate Transition2/1
  Rate Transition2/1 -> Out1/1

== system PPS_Model/PPS Model/Actuation/Braking Lights ==
  note: === Braking lights block ===
      |
      |    - according to brake pressure, lights up braking lights of the actor,
      |    - the signal is a 3x1 vector:
      |      = first        value - left braking light,
      |      = second value - middle braking light,
      |      = third       value - right braking light.
  switcher : Inport
  Add : Sum
  Constant : Constant
  Constant1 : Constant  Value=0
  Mux : Mux  Inputs=3
  Pulse Generator : DiscretePulseGenerator  PulseType=Time based  Period=0.6  PulseWidth=50  PhaseDelay=0.3
  Rate Transition3 : RateTransition  Integrity=off  Deterministic=off  OutPortSampleTime=[0,0]
  Switch : Switch  Criteria=u2 > Threshold
  Switch1 : Switch  Criteria=u2 > Threshold
  Switch2 : Switch  Criteria=u2 > Threshold
  Unary Minus : UnaryMinus
  BrakeLights (3x1) : Outport
  wires:
  Mux/1 -> BrakeLights (3x1)/1
  switcher/1 -> Switch/2, Switch1/2, Switch2/2
  Constant/1 -> Switch/1, Add/2
  Switch/1 -> Switch1/3, Switch2/3, Mux/2
  Constant1/1 -> Switch/3
  Switch2/1 -> Mux/1
  Switch1/1 -> Mux/3
  Pulse Generator/1 -> Rate Transition3/1
  Add/1 -> Switch1/1
  Unary Minus/1 -> Add/1
  Rate Transition3/1 -> Unary Minus/1, Switch2/1

== system PPS_Model/PPS Model/Actuation/If Action Subsystem ==
  Action Port : ActionPort  ActionType=then
  Constant1 : Constant  SampleTime=[0,0]
  Data Store Write : DataStoreWrite  DataStoreName=full_brake
  wires:
  Constant1/1 -> Data Store Write/1

== system PPS_Model/PPS Model/PPS EGO State Display/Display function ==
  V [km/h] : Inport
  RPM : Inport  Port=2
  Brake Pressure : Inport  Port=3
  Detection flag : Inport  Port=4
  Warning Flag : Inport  Port=5
  Braking flag : Inport  Port=6
  Pet det flag : Inport  Port=7
  TTC : Inport  Port=8
  Enable : EnablePort
  Brake Pressure [bar]2 : Gain  Gain=100/MaxBrakePressure
  EGO Vehicle state display : M-S-Function  FunctionName=msfcn_PPS_PlotSpeed  Parameters=DisplayFreq DisplaySwitch
  Rounding Function2 : Rounding  Operator=round
  Rounding Function3 : Rounding  Operator=round
  wires:
  Brake Pressure [bar]2/1 -> Rounding Function3/1
  Rounding Function3/1 -> EGO Vehicle state display/3
  Rounding Function2/1 -> EGO Vehicle state display/2
  V [km/h]/1 -> EGO Vehicle state display/1
  Detection flag/1 -> EGO Vehicle state display/4
  Warning Flag/1 -> EGO Vehicle state display/5
  Braking flag/1 -> EGO Vehicle state display/6
  Pet det flag/1 -> EGO Vehicle state display/7
  TTC/1 -> EGO Vehicle state display/8
  RPM/1 -> Rounding Function2/1
  Brake Pressure/1 -> Brake Pressure [bar]2/1

== system PPS_Model/PPS Model/PPS EGO State Display/Plots ==
  V : Inport
  Ax : Inport  Port=2  SampleTime=[0,0]
  det : Inport  Port=3
  warn : Inport  Port=4
  brake : Inport  Port=5
  ped : Inport  Port=6
  ttc : Inport  Port=7
  Constant : Constant  Value=0
  Data Type Conversion4 : DataTypeConversion  OutDataTypeStr=double
  Mux : Mux
  Mux1 : Mux
  Rate Transition5 : RateTransition  Integrity=off  OutPortSampleTime=1/DisplayFreq
  Switch1 : Switch  Threshold=4
  To Workspace2 : ToWorkspace  VariableName=VRU_simout  SampleTime=0.04  SaveFormat=Structure With Time
  wires:
  Mux/1 -> To Workspace2/1
  Mux1/1 -> Data Type Conversion4/1
  Data Type Conversion4/1 -> Mux/3
  Ax/1 -> Rate Transition5/1
  Rate Transition5/1 -> Mux/2
  Switch1/1 -> Mux/4
  Constant/1 -> Switch1/1
  V/1 -> Mux/1
  det/1 -> Mux1/1
  warn/1 -> Mux1/2
  brake/1 -> Mux1/3
  ped/1 -> Mux1/4
  ttc/1 -> Switch1/2, Switch1/3

== system PPS_Model/PPS Model/PPS_Radar/Radar ==
  Range : Inport
  Theta : Inport  Port=2
  All flags : Inport  Port=3
  Flag 0.6 : Inport  Port=4
  Enable : EnablePort
  DISPLAY1 : M-S-Function  FunctionName=msfcn_PPS_radar_graph  Parameters=RadarFreq TISdet RadarSwitch TISMaxRange TISMaxTheta*pi/180
  Degrees to Radians : simulink_extras/Transformations/Degrees to Radians  SystemSampleTime=-1
  wires:
  Range/1 -> DISPLAY1/1
  Theta/1 -> Degrees to Radians/1
  All flags/1 -> DISPLAY1/3
  Flag 0.6/1 -> DISPLAY1/4
  Degrees to Radians/1 -> DISPLAY1/2

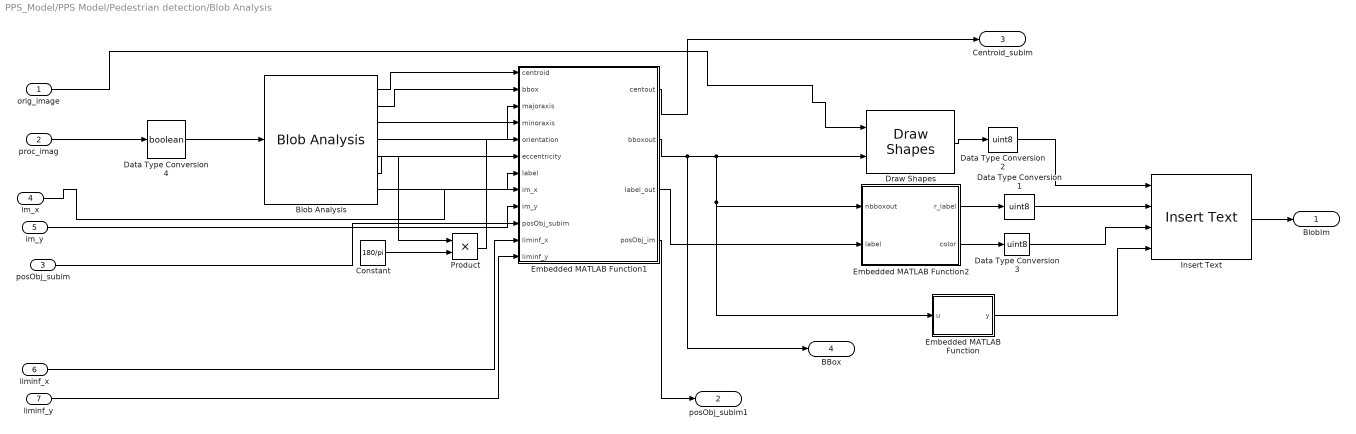
== system PPS_Model/PPS Model/Pedestrian detection/Blob Analysis ==
  orig_image : Inport
  proc_imag : Inport  Port=2
  posObj_subim : Inport  Port=3
  im_x : Inport  Port=4
  im_y : Inport  Port=5
  liminf_x : Inport  Port=6
  liminf_y : Inport  Port=7
  Blob Analysis : vipstatistics/Blob Analysis  Tag=vipblks_row_conv  DialogController=vipDDGCreate  DialogControllerArgs=DataTag1  area=off  centroid=on  bBox=on  majorAxis=on  minorAxis=on  angle=on  eccentricity=on  equivDiameterSq=off  extent=off  perimeter=off  maxBlobs=100  warnIfNumBlobsExceeded=on  isCount=off  useMinArea=on  minArea=50  useMaxArea=on  maxArea=150000  excludeBorderBlob=off  outDT=single  isOutVarDim=off  isFill=on  fillValues=-1  conn=4  isLabel=on  outputMode=Binary point scaling  outputWordLength=32  outputFracLength=16  firstCoeffMode=Binary point scaling  firstCoeffWordLength=16  firstCoeffFracLength=14  secondCoeffMode=Binary point scaling  secondCoeffWordLength=32  secondCoeffFracLength=16  accumMode=Binary point scaling  accumWordLength=32  accumFracLength=0  prodOutputMode=Binary point scaling  prodOutputWordLength=32  prodOutputFracLength=16  roundingMode=Floor  overflowMode=off
  Constant : Constant  Value=180/pi  VectorParams1D=off
  Data Type Conversion1 : DataTypeConversion  OutDataTypeStr=uint8
  Data Type Conversion2 : DataTypeConversion  OutDataTypeStr=uint8
  Data Type Conversion3 : DataTypeConversion  OutDataTypeStr=uint8
  Data Type Conversion4 : DataTypeConversion  OutDataTypeStr=boolean
  Draw Shapes : viptextngfix/Draw Shapes  DialogController=vipDDGCreate  DialogControllerArgs=DataTag2  shape=Rectangles  fill=off  fillClrSource=Specify via dialog  display=White  intensity=200  color=[200 255 100]  opacity=0.4  viewport=Entire image  antialiasing=off  inType=Obsolete  imagePorts=One multidimensional signal  prodOutputMode=Binary point scaling  prodOutputWordLength=32  prodOutputFracLength=14  memoryMode=Specify word length  memoryWordLength=16  memoryFracLength=14  roundingMode=Floor  overflowMode=off
  Embedded MATLAB Function : Stateflow chart  TreatAsAtomicUnit=on
  Embedded MATLAB Function1 : Stateflow chart  TreatAsAtomicUnit=on
  Embedded MATLAB Function2 : Stateflow chart  TreatAsAtomicUnit=on
  Insert Text : viptextngfix/Insert Text  DialogController=vipDDGCreate  DialogControllerArgs=DataTag3  inputType=Obsolete  theText='%02d'  fontFace=LucidaSansRegular  dummyVar1=0  blockFontSize=12  antiAliased=on  getTextLocFrom=Input port  textLoc=[0 0]  getTextColorFrom=Input port  textColor=zeros(1,size(nbboxout,2))  getTextIntensityFrom=Specify via dialog  textIntensity=0  getTextOpacityFrom=Specify via dialog  textOpacity=1.0  dummyVar2=0  dummyVar3=0  dummyVar4=0  imagePorts=One multidimensional signal  isInputTransposed=off
  Product : Product  RndMeth=Zero
  BlobIm : Outport
  posObj_subim1 : Outport  Port=2
  Centroid_subim : Outport  Port=3
  BBox : Outport  Port=4
  wires:
  Blob Analysis/4 -> Embedded MATLAB Function1/4(minoraxis)
  Constant/1 -> Product/2
  Embedded MATLAB Function2/1(r_label) -> Data Type Conversion1/1
  Embedded MATLAB Function2/2(color) -> Data Type Conversion3/1
  Draw Shapes/1 -> Data Type Conversion2/1
  Data Type Conversion1/1 -> Insert Text/2
  Data Type Conversion2/1 -> Insert Text/1
  Data Type Conversion3/1 -> Insert Text/3
  Blob Analysis/1 -> Embedded MATLAB Function1/1(centroid)
  Blob Analysis/2 -> Embedded MATLAB Function1/2(bbox)
  Blob Analysis/3 -> Embedded MATLAB Function1/3(majoraxis)
  Blob Analysis/5 -> Product/1
  Product/1 -> Embedded MATLAB Function1/5(orientation)
  Blob Analysis/6 -> Embedded MATLAB Function1/6(eccentricity)
  Blob Analysis/7 -> Embedded MATLAB Function1/7(label)
  Embedded MATLAB Function1/3(label_out) -> Embedded MATLAB Function2/2(label)
  Embedded MATLAB Function1/2(bboxout) -> Draw Shapes/2, Embedded MATLAB Function2/1(nbboxout), Embedded MATLAB Function/1(u), BBox/1
  Embedded MATLAB Function1/1(centout) -> Centroid_subim/1
  Insert Text/1 -> BlobIm/1
  proc_imag/1 -> Data Type Conversion4/1
  im_x/1 -> Embedded MATLAB Function1/8(im_x)
  orig_image/1 -> Draw Shapes/1
  im_y/1 -> Embedded MATLAB Function1/9(im_y)
  liminf_x/1 -> Embedded MATLAB Function1/11(liminf_x)
  liminf_y/1 -> Embedded MATLAB Function1/12(liminf_y)
  posObj_subim/1 -> Embedded MATLAB Function1/10(posObj_subim)
  Embedded MATLAB Function1/4(posObj_im) -> posObj_subim1/1
  Data Type Conversion4/1 -> Blob Analysis/1
  Embedded MATLAB Function/1(y) -> Insert Text/4

== system PPS_Model/PPS Model/Pedestrian detection/Image processing ==
  Image : Inport
  Closing : vipmorphops/Closing  nhoodsrc=Specify via dialog  strel=strel('disk', 4)
  Edge Detection : vipanalysis/Edge Detection  DialogController=vipDDGCreate  DialogControllerArgs=DataTag17  method=Canny  outputType=Binary image  userDefinedThreshold=off  thresholdSource=Specify via dialog  threshold=1  thresholdTuning=3  edgeThinning=off  threshold_canny=[0.25 0.60]  autoPercent=93  sigma=1  prodOutputMode=Binary point scaling  prodOutputWordLength=32  prodOutputFracLength=8  roundingMode=Floor  overflowMode=off
  Embedded MATLAB Function : Stateflow chart  TreatAsAtomicUnit=on
  Image Data Type Conversion1 : vipconversions/Image Data Type Conversion  outDT=single  isSigned=on  wordLen=16  numFracBits=0
  ProcIm : Outport
  wires:
  Closing/1 -> Embedded MATLAB Function/1(image)
  Embedded MATLAB Function/1(im) -> ProcIm/1
  Image/1 -> Image Data Type Conversion1/1
  Edge Detection/1 -> Closing/1
  Image Data Type Conversion1/1 -> Edge Detection/1

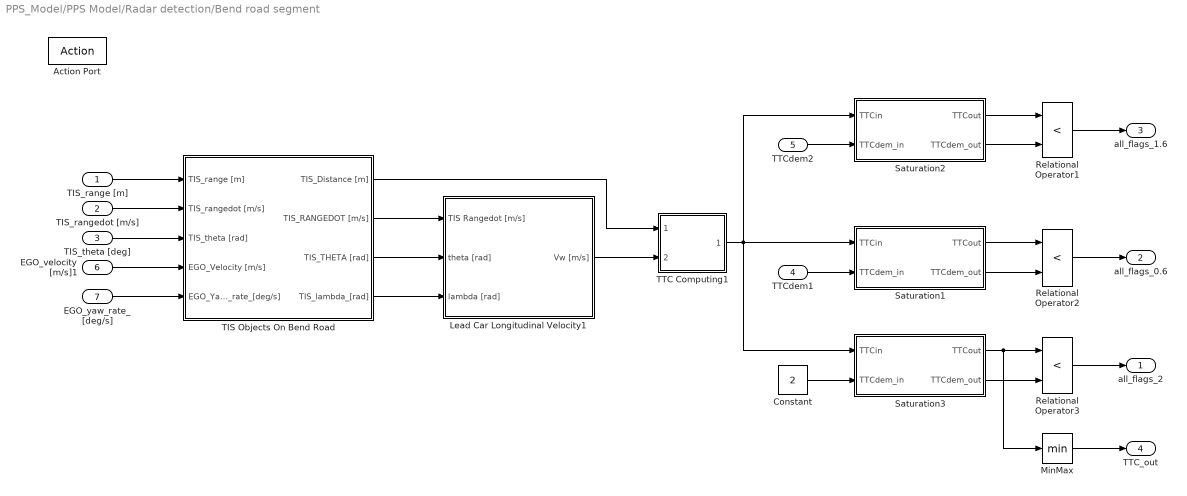
== system PPS_Model/PPS Model/Radar detection/Bend road segment ==
  TIS_range [m] : Inport  PortDimensions=TISdet
  TIS_rangedot [m/s] : Inport  Port=2  PortDimensions=TISdet
  TIS_theta [deg] : Inport  Port=3  PortDimensions=TISdet
  TTCdem1 : Inport  Port=4
  TTCdem2 : Inport  Port=5
  EGO_velocity [m/s]1 : Inport  Port=6
  EGO_yaw_rate_[deg/s] : Inport  Port=7
  Action Port : ActionPort  ActionType=then
  Constant : Constant  Value=2
  Lead Car Longitudinal Velocity1 : Subsystem
  MinMax : MinMax
  Relational Operator1 : RelationalOperator  Operator=<  OutDataTypeStr=fixdt(1,16)
  Relational Operator2 : RelationalOperator  Operator=<  OutDataTypeStr=fixdt(1,16)
  Relational Operator3 : RelationalOperator  Operator=<  OutDataTypeStr=fixdt(1,16)
  Saturation1 : Subsystem
  Saturation2 : Subsystem
  Saturation3 : Subsystem
  TIS Objects On Bend Road : Subsystem
  TTC Computing1 : Subsystem
  all_flags_2 : Outport  InitialOutput=0
  all_flags_0.6 : Outport  Port=2  InitialOutput=0
  all_flags_1.6 : Outport  Port=3  InitialOutput=zeros(TISdet,1)
  TTC_out : Outport  Port=4
  wires:
  EGO_yaw_rate_[deg/s]/1 -> TIS Objects On Bend Road/5(EGO_Yaw_rate_[deg/s])
  Lead Car Longitudinal Velocity1/1(Vw [m/s]) -> TTC Computing1/2(Velocity [m/s])
  EGO_velocity [m/s]1/1 -> TIS Objects On Bend Road/4(EGO_Velocity [m/s])
  TIS Objects On Bend Road/1(TIS_Distance [m]) -> TTC Computing1/1(Distance [m])
  TIS Objects On Bend Road/2(TIS_RANGEDOT [m/s]) -> Lead Car Longitudinal Velocity1/1(TIS Rangedot [m/s])
  TIS Objects On Bend Road/3(TIS_THETA [rad]) -> Lead Car Longitudinal Velocity1/2(theta [rad])
  TIS Objects On Bend Road/4(TIS_lambda_[rad]) -> Lead Car Longitudinal Velocity1/3(lambda [rad])
  TIS_range [m]/1 -> TIS Objects On Bend Road/1(TIS_range [m])
  TIS_rangedot [m/s]/1 -> TIS Objects On Bend Road/2(TIS_rangedot [m/s])
  TIS_theta [deg]/1 -> TIS Objects On Bend Road/3(TIS_theta [rad])
  TTC Computing1/1(TTC [s]) -> Saturation3/1(TTCin), Saturation1/1(TTCin), Saturation2/1(TTCin)
  Saturation2/1(TTCout) -> Relational Operator1/1
  Relational Operator1/1 -> all_flags_1.6/1
  TTCdem2/1 -> Saturation2/2(TTCdem_in)
  Saturation2/2(TTCdem_out) -> Relational Operator1/2
  Relational Operator2/1 -> all_flags_0.6/1
  TTCdem1/1 -> Saturation1/2(TTCdem_in)
  Saturation1/1(TTCout) -> Relational Operator2/1
  Saturation1/2(TTCdem_out) -> Relational Operator2/2
  MinMax/1 -> TTC_out/1
  Constant/1 -> Saturation3/2(TTCdem_in)
  Saturation3/2(TTCdem_out) -> Relational Operator3/2
  Saturation3/1(TTCout) -> Relational Operator3/1, MinMax/1
  Relational Operator3/1 -> all_flags_2/1

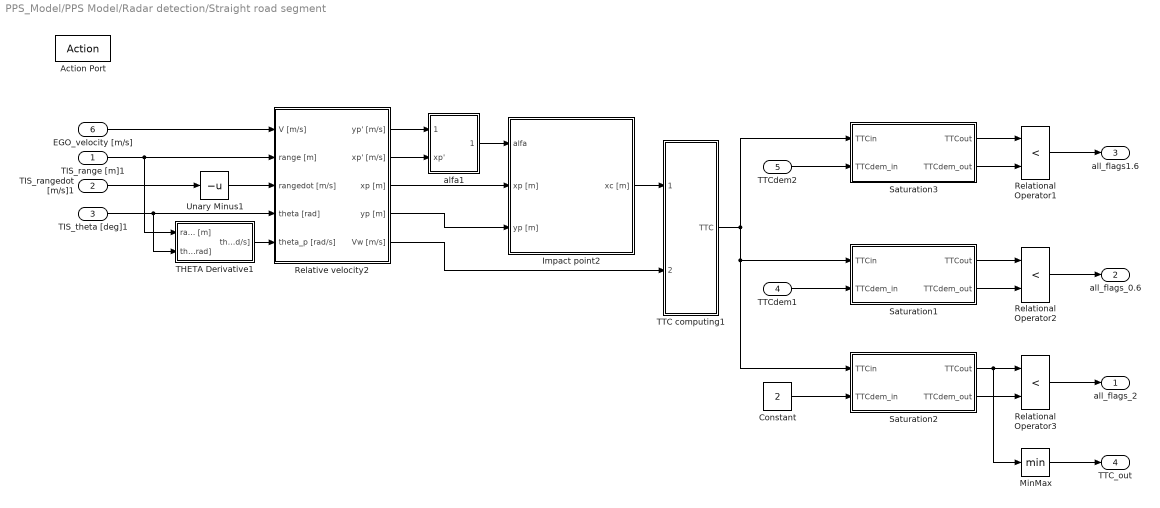
== system PPS_Model/PPS Model/Radar detection/Straight road segment ==
  TIS_range [m]1 : Inport  PortDimensions=TISdet
  TIS_rangedot [m/s]1 : Inport  Port=2  PortDimensions=TISdet
  TIS_theta [deg]1 : Inport  Port=3  PortDimensions=TISdet
  TTCdem1 : Inport  Port=4
  TTCdem2 : Inport  Port=5
  EGO_velocity [m/s] : Inport  Port=6
  Action Port : ActionPort  ActionType=else
  Constant : Constant  Value=2
  Impact point2 : Subsystem
  MinMax : MinMax
  Relational Operator1 : RelationalOperator  Operator=<  OutDataTypeStr=fixdt(1,16)
  Relational Operator2 : RelationalOperator  Operator=<  OutDataTypeStr=fixdt(1,16)
  Relational Operator3 : RelationalOperator  Operator=<  OutDataTypeStr=fixdt(1,16)
  Relative velocity2 : Subsystem
  Saturation1 : Subsystem
  Saturation2 : Subsystem
  Saturation3 : Subsystem
  THETA Derivative1 : Subsystem
  TTC computing1 : Subsystem
  Unary Minus1 : UnaryMinus
  alfa1 : Subsystem
  all_flags_2 : Outport  InitialOutput=0
  all_flags_0.6 : Outport  Port=2  SampleTime=1/TISfreq  InitialOutput=0
  all_flags1.6 : Outport  Port=3  SampleTime=1/TISfreq  InitialOutput=0
  TTC_out : Outport  Port=4
  wires:
  EGO_velocity [m/s]/1 -> Relative velocity2/1(V [m/s])
  TIS_range [m]1/1 -> THETA Derivative1/1(range [m]), Relative velocity2/2(range [m])
  TIS_rangedot [m/s]1/1 -> Unary Minus1/1
  TIS_theta [deg]1/1 -> Relative velocity2/4(theta [rad]), THETA Derivative1/2(theta [rad])
  THETA Derivative1/1(theta_dot [rad/s]) -> Relative velocity2/5(theta_p [rad/s])
  Relative velocity2/1(yp' [m/s]) -> alfa1/1(yp'1)
  Relative velocity2/2(xp' [m/s]) -> alfa1/2(xp')
  Relative velocity2/3(xp [m]) -> Impact point2/2(xp [m])
  alfa1/1(alfa1) -> Impact point2/1(alfa)
  Unary Minus1/1 -> Relative velocity2/3(rangedot [m/s])
  Relative velocity2/4(yp [m]) -> Impact point2/3(yp [m])
  Impact point2/1(xc [m]) -> TTC computing1/1(xc [m])
  Relative velocity2/5(Vw [m/s]) -> TTC computing1/2(Vw [m/s])
  TTC computing1/1(TTC) -> Saturation1/1(TTCin), Saturation2/1(TTCin), Saturation3/1(TTCin)
  Saturation3/1(TTCout) -> Relational Operator1/1
  Relational Operator1/1 -> all_flags1.6/1
  TTCdem2/1 -> Saturation3/2(TTCdem_in)
  Saturation3/2(TTCdem_out) -> Relational Operator1/2
  Relational Operator2/1 -> all_flags_0.6/1
  TTCdem1/1 -> Saturation1/2(TTCdem_in)
  Saturation1/1(TTCout) -> Relational Operator2/1
  Saturation1/2(TTCdem_out) -> Relational Operator2/2
  Constant/1 -> Saturation2/2(TTCdem_in)
  Saturation2/2(TTCdem_out) -> Relational Operator3/2
  Saturation2/1(TTCout) -> Relational Operator3/1, MinMax/1
  Relational Operator3/1 -> all_flags_2/1
  MinMax/1 -> TTC_out/1
